simulink model "sampleModel197"  (R2021b)
settings: Solver=VariableStepAuto  StartTime=0.0  StopTime=10.0  RelTol=1e-3
undefined symbols (not defined in the file or in its folder): Newton, Raphson
libraries: simulink x2, slpidlib x1
settings Model: Creator=user  LastModifiedBy=user

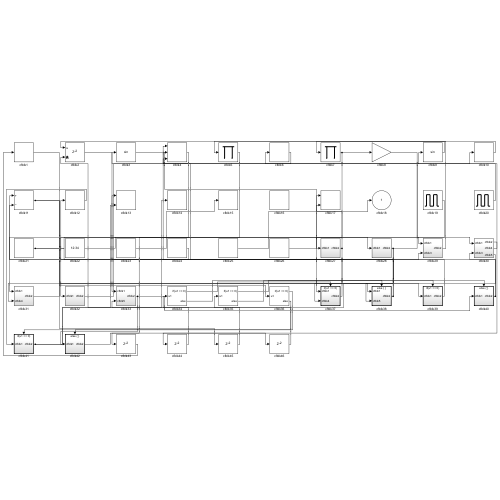
[thumbnail: Simulink's stored preview of the top-level diagram]
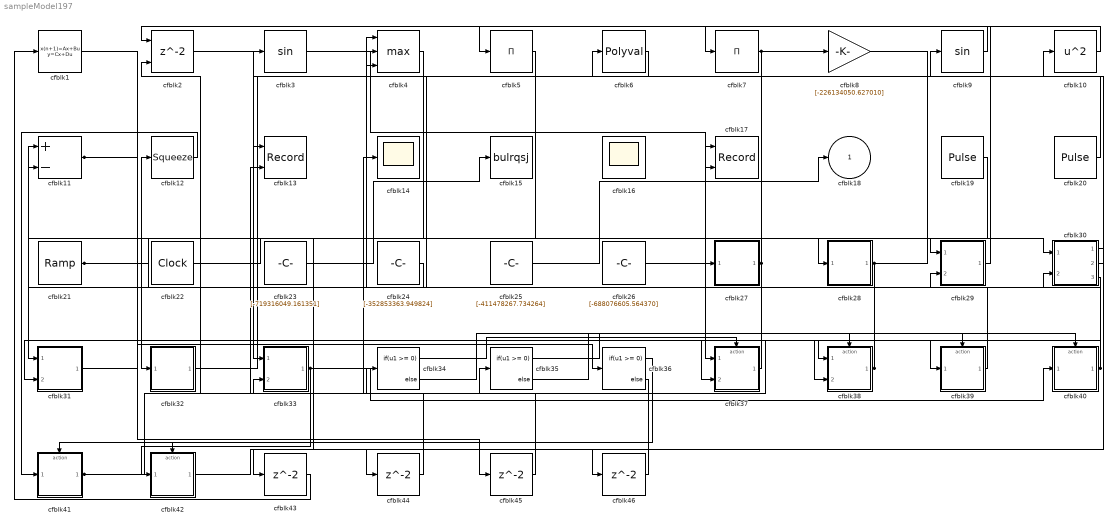
== system sampleModel197 ==
  cfblk1 : DiscreteStateSpace
  cfblk10 : Math  Operator=square  SaturateOnIntegerOverflow=on
  cfblk11 : Sum  Inputs=+-
  cfblk12 : Squeeze
  cfblk13 : Record  FileSettingsInternal="{\"entries\":[{\"content\":{\"excelSettings\":{\"content\":{},\"type\":\"Streamout.ExcelSettings\"}},\"type\":\"Streamout.FileSettingStorage\",\"uuid\":\"0279d5a8-bec8-47d0-96a9-0591946e5d00\"}],\"packageUris\":[\"http://schema.mathworks.com/mf0/streamout_blocks/R2020a\"],\"version\":\"1.0\"}"  Layout=[1 1]  SignalsInternal="{\"entries\":[{\"content\":{\"signals\":[{\"content\":{\"blockPath\":[\"sampleModel197/cfblk13\"],\"channel\":[],\"dimensions\":[1],\"domain\":\"sampleModel197/cfblk13\",\"lineColor\":\"#a2142f\",\"plots\":[1],\"port\":1,\"sid\":[\"\"],\"signalID\":7568,\"signalName\":\"cfblk40\"},\"type\":\"RecordBlkView.Signal\",\"uuid\":\"e7f566aa-51c7-4da6-b2fc-9a33eccfc797\"},{\"content\":{\"blockPath\":[\"sampleModel197/cfblk13\"],\"channel\":[],\"dimensions\":[1],\"domain\":\"sampleModel197/cfblk13\",\"lineColor\":\"#139fff\",\"plots\":[1],\"port\":2,\"sid\":[\"\"],\"signalID\":7572,\"signalName\":\"cfblk41\"},\"type\":\"RecordBlkView.Signal\",\"uuid\":\"1b39f455-c7ec-4c6a-a985-f4122d27351c\"}]},\"type\":\"RecordBlkView.InputSignals\",\"uuid\":\"b38396f4-be78-40d0-b78e-78bdf6d546fb\"}],\"packageUris\":[\"http://schema.mathworks.com/mf0/streamout_blocks/R2020a\"],\"version\":\"1.0\"}"  VisualizationBindings="{\"xyplotplugin\":{\"info\":[{\"series\":[{\"bindingParametersList\":[{\"parameter\":\"X-Axis\",\"signalID\":7568,\"signalName\":\"cfblk40\"},{\"parameter\":\"Y-Axis\",\"signalID\":7572,\"signalName\":\"cfblk41\"}],\"seriesID\":61193}],\"subplotID\":1}]}}"  CompatibilityTag=XY
  cfblk14 : Scope
  cfblk15 : ToWorkspace  VariableName=bulrqsj  SaveFormat=Timeseries  SampleTime=-1
  cfblk16 : Scope
      settings: Floating=on
  cfblk17 : Record  FileSettingsInternal="{\"entries\":[{\"content\":{\"excelSettings\":{\"content\":{},\"type\":\"Streamout.ExcelSettings\"}},\"type\":\"Streamout.FileSettingStorage\",\"uuid\":\"e6ae8cde-df67-4d7c-a82d-89148d2c1f8a\"}],\"packageUris\":[\"http://schema.mathworks.com/mf0/streamout_blocks/R2020a\"],\"version\":\"1.0\"}"  Layout=[1 1]  SignalsInternal="{\"entries\":[{\"content\":{\"signals\":[{\"content\":{\"blockPath\":[\"sampleModel197/cfblk17\"],\"channel\":[],\"dimensions\":[1],\"domain\":\"sampleModel197/cfblk17\",\"lineColor\":\"#a2142f\",\"plots\":[1],\"port\":1,\"sid\":[\"\"],\"signalID\":7576,\"signalName\":\"cfblk27\"},\"type\":\"RecordBlkView.Signal\",\"uuid\":\"cf26e29d-c82c-4e0b-80be-766500b7eef1\"},{\"content\":{\"blockPath\":[\"sampleModel197/cfblk17\"],\"channel\":[],\"dimensions\":[1],\"domain\":\"sampleModel197/cfblk17\",\"lineColor\":\"#139fff\",\"plots\":[1],\"port\":2,\"sid\":[\"\"],\"signalID\":7580,\"signalName\":\"cfblk26\"},\"type\":\"RecordBlkView.Signal\",\"uuid\":\"675d0609-db64-4a86-b5a2-412efc60ee90\"}]},\"type\":\"RecordBlkView.InputSignals\",\"uuid\":\"0deeecff-eec2-4d60-b210-f9e7a71af17f\"}],\"packageUris\":[\"http://schema.mathworks.com/mf0/streamout_blocks/R2020a\"],\"version\":\"1.0\"}"  VisualizationBindings="{\"xyplotplugin\":{\"info\":[{\"series\":[{\"bindingParametersList\":[{\"parameter\":\"X-Axis\",\"signalID\":7576,\"signalName\":\"cfblk27\"},{\"parameter\":\"Y-Axis\",\"signalID\":7580,\"signalName\":\"cfblk26\"}],\"seriesID\":48152}],\"subplotID\":1}]}}"  CompatibilityTag=XY
  cfblk19 : DiscretePulseGenerator  PulseType=Time based  Amplitude=[213944158.153628]  Period=[64533026.569931]  PulseWidth=5  PhaseDelay=[3.000000]
  cfblk2 : Delay  ShowEnablePort=on  SampleTime=1
      settings: InputPortMap=u0,e6
  cfblk20 : DiscretePulseGenerator  PulseType=Time based  Amplitude=[999071178.653989]  Period=[57734423.716283]  PulseWidth=5  PhaseDelay=[7.000000]
  cfblk21 : simulink/Sources/Ramp  slope=[-9275.531510]  start=[11.118864]  InitialOutput=[640340.774818]
  cfblk22 : DigitalClock
  cfblk23 : Constant  Value=[-719316049.161351]  SampleTime=1
  cfblk24 : Constant  Value=[-352853363.949824]  SampleTime=1
  cfblk25 : Constant  Value=[-411478267.734264]  SampleTime=1
  cfblk26 : Constant  Value=[-688076605.564370]  SampleTime=1
  cfblk27 : Subsystem
  cfblk28 : Subsystem
  cfblk29 : Subsystem
  cfblk3 : Trigonometry
  cfblk30 : Subsystem
  cfblk31 : Subsystem
  cfblk32 : Subsystem
  cfblk33 : Subsystem
  cfblk34 : If  IfExpression=u1 >= 0  SampleTime=1
  cfblk35 : If  IfExpression=u1 >= 0  SampleTime=1
  cfblk36 : If  IfExpression=u1 >= 0  SampleTime=1
  cfblk37 : Subsystem  TreatAsAtomicUnit=on
  cfblk38 : Subsystem  TreatAsAtomicUnit=on
  cfblk39 : Subsystem  TreatAsAtomicUnit=on
  cfblk4 : MinMax  Function=max  Inputs=3
  cfblk40 : Subsystem  TreatAsAtomicUnit=on
  cfblk41 : Subsystem  TreatAsAtomicUnit=on
  cfblk42 : Subsystem  TreatAsAtomicUnit=on
  cfblk{43..46} (4 alike) : Delay  SampleTime=1
  cfblk5 : Product  Inputs=*
  cfblk6 : Polyval  Coefs=[ +2.081618890e-019, -1.441693666e-014, +4.719686976e-010, -8.536869453e-006, +1.621573104e-001, -8.087801117e+001 ]
  cfblk7 : Product  Inputs=*
  cfblk8 : Gain  Gain=[-226134050.627010]
  cfblk9 : Trigonometry
  cfblk18 : Outport
  wires:
  cfblk23/1 -> cfblk15/1
  cfblk3/1 -> cfblk37/1(cfblk1)
  cfblk28/1(cfblk2) -> cfblk35/1, cfblk10/1, cfblk38/2(cfblk5)
  cfblk24/1 -> cfblk11/1
  cfblk33/1(cfblk2) -> cfblk40/1(cfblk1), cfblk42/1(cfblk1)
  cfblk37/1(cfblk2) -> cfblk11/2
  cfblk32/1(cfblk2) -> cfblk9/1
  cfblk11/1 -> cfblk36/1, cfblk45/1
  cfblk25/1 -> cfblk18/1
  cfblk2/1 -> cfblk33/1(cfblk1)
  cfblk7/1 -> cfblk8/1, cfblk31/1(cfblk1)
  cfblk27/1(cfblk2) -> cfblk17/1, cfblk31/2(cfblk4)
  cfblk12/1 -> cfblk41/1(cfblk1)
  cfblk29/1(cfblk2) -> cfblk5/1
  cfblk26/1 -> cfblk17/2
  cfblk10/1 -> cfblk7/1
  cfblk20/1 -> cfblk3/1
  cfblk39/1(cfblk2) -> cfblk4/1
  cfblk9/1 -> cfblk2/1
  cfblk5/1 -> cfblk32/1(cfblk1)
  cfblk21/1 -> cfblk29/1(cfblk1), cfblk29/2(cfblk3)
  cfblk41/1(cfblk2) -> cfblk14/1, cfblk13/2
  cfblk22/1 -> cfblk28/1(cfblk1)
  cfblk40/1(cfblk2) -> cfblk13/1, cfblk30/2(cfblk3)
  cfblk8/1 -> cfblk30/1(cfblk1)
  cfblk19/1 -> cfblk27/1(cfblk1)
  cfblk6/1 -> cfblk4/2
  cfblk1/1 -> cfblk39/1(cfblk1)
  cfblk30/2(cfblk4) -> cfblk6/1
  cfblk31/1(cfblk2) -> cfblk38/1(cfblk1)
  cfblk30/3(cfblk5) -> cfblk37/2(cfblk4)
  cfblk38/1(cfblk2) -> cfblk12/1, cfblk4/3
  cfblk34/1 -> cfblk37/Action
  cfblk34/2 -> cfblk38/Action
  cfblk35/1 -> cfblk39/Action
  cfblk35/2 -> cfblk40/Action
  cfblk36/1 -> cfblk41/Action
  cfblk36/2 -> cfblk42/Action
  cfblk4/1 -> cfblk43/1
  cfblk43/1 -> cfblk1/1
  cfblk30/1(cfblk2) -> cfblk44/1
  cfblk44/1 -> cfblk2/2
  cfblk45/1 -> cfblk34/1
  cfblk42/1(cfblk2) -> cfblk46/1
  cfblk46/1 -> cfblk33/2(cfblk5)

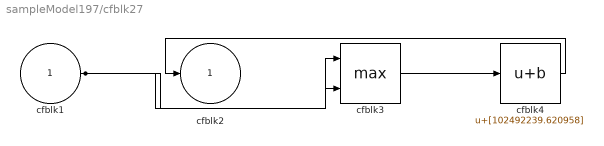
== system sampleModel197/cfblk27 ==
  cfblk1 : Inport
  cfblk3 : MinMax  Function=max  Inputs=2
  cfblk4 : Bias  Bias=[102492239.620958]
  cfblk2 : Outport
  wires:
  cfblk4/1 -> cfblk2/1
  cfblk3/1 -> cfblk4/1
  cfblk1/1 -> cfblk3/1, cfblk3/2

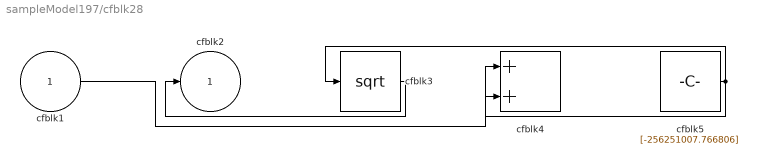
== system sampleModel197/cfblk28 ==
  cfblk1 : Inport
  cfblk3 : Sqrt  SaturateOnIntegerOverflow=on
  cfblk4 : Sum
  cfblk5 : Constant  Value=[-256251007.766806]  SampleTime=1
  cfblk2 : Outport
  wires:
  cfblk5/1 -> cfblk3/1, cfblk4/2
  cfblk3/1 -> cfblk2/1
  cfblk1/1 -> cfblk4/1

== system sampleModel197/cfblk29 ==
  cfblk1 : Inport
  cfblk3 : Inport  Port=2
  cfblk2 : Outport
  wires:
  cfblk1/1 -> cfblk2/1

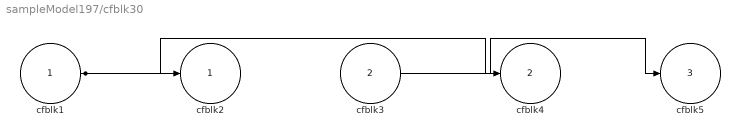
== system sampleModel197/cfblk30 ==
  cfblk1 : Inport
  cfblk3 : Inport  Port=2
  cfblk2 : Outport
  cfblk4 : Outport  Port=2
  cfblk5 : Outport  Port=3
  wires:
  cfblk3/1 -> cfblk5/1
  cfblk1/1 -> cfblk2/1, cfblk4/1

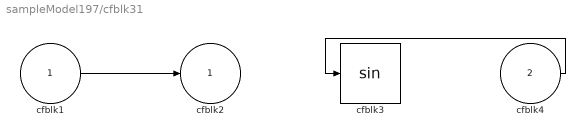
== system sampleModel197/cfblk31 ==
  cfblk1 : Inport
  cfblk4 : Inport  Port=2
  cfblk3 : Trigonometry
  cfblk2 : Outport
  wires:
  cfblk1/1 -> cfblk2/1
  cfblk4/1 -> cfblk3/1

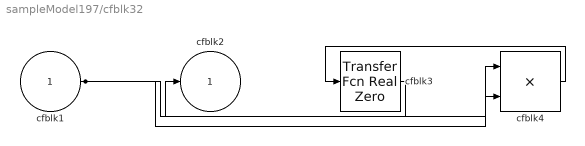
== system sampleModel197/cfblk32 ==
  cfblk1 : Inport
  cfblk3 : simulink/Discrete/Transfer Fcn Real Zero  ZeroZ=0.75  ICPrevInput=0.0  DoSatur=off
      settings: SourceProductBaseCode=SL
  cfblk4 : Product  Inputs=**
  cfblk2 : Outport
  wires:
  cfblk4/1 -> cfblk3/1
  cfblk3/1 -> cfblk2/1
  cfblk1/1 -> cfblk4/1, cfblk4/2

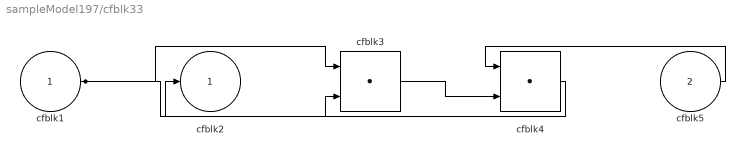
== system sampleModel197/cfblk33 ==
  cfblk1 : Inport
  cfblk5 : Inport  Port=2
  cfblk3 : DotProduct  InputSameDT=on  OutDataTypeStr=Inherit: Inherit via internal rule
  cfblk4 : DotProduct  InputSameDT=on  OutDataTypeStr=Inherit: Inherit via internal rule
  cfblk2 : Outport
  wires:
  cfblk5/1 -> cfblk4/1
  cfblk3/1 -> cfblk4/2
  cfblk4/1 -> cfblk2/1
  cfblk1/1 -> cfblk3/1, cfblk3/2

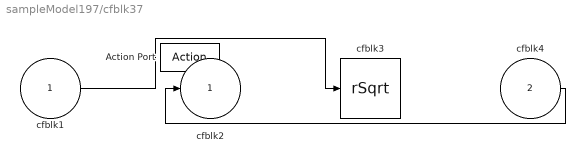
== system sampleModel197/cfblk37 ==
  cfblk1 : Inport
  cfblk4 : Inport  Port=2
  Action Port : ActionPort  ActionPortLabel=if(u1 >= 0)
  cfblk3 : Sqrt  Operator=rSqrt  AlgorithmType=Newton-Raphson  SaturateOnIntegerOverflow=on
  cfblk2 : Outport
  wires:
  cfblk4/1 -> cfblk2/1
  cfblk1/1 -> cfblk3/1

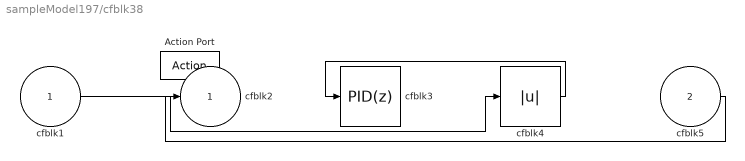
== system sampleModel197/cfblk38 ==
  cfblk1 : Inport
  cfblk5 : Inport  Port=2
  Action Port : ActionPort  ActionPortLabel=else
  cfblk3 : slpidlib/PID Controller  Controller=PID  Form=Parallel  TimeDomain=Discrete-time  UseExternalTs=off  SampleTime=-1  IntegratorMethod=Forward Euler  FilterMethod=Forward Euler  ControllerParametersSource=internal  P=1  I=1  D=0  UseFilter=on  N=100  TunerSelectOption=Transfer Function Based (PID Tuner App)  InitialConditionSource=internal  InitialConditionForIntegrator=0  InitialConditionForFilter=0  DifferentiatorICPrevScaledInput=0  ExternalReset=none  TrackingMode=off  Kt=1  LimitOutput=off  SatLimitsSource=internal  UpperSaturationLimit=inf  LowerSaturationLimit=-inf  LinearizeAsGain=off  AntiWindupMode=none  Kb=1  POutMin=[]  POutMax=[]  IOutMin=[]  IOutMax=[]  DOutMin=[]  DOutMax=[]  NOutMin=[]  NOutMax=[]  SumOutMin=[]  SumOutMax=[]  SaturationOutMin=[]  SaturationOutMax=[]  PParamMin=[]  PParamMax=[]  IParamMin=[]  IParamMax=[]  DParamMin=[]  DParamMax=[]  NParamMin=[]  NParamMax=[]  KbParamMin=[]  KbParamMax=[]  KtParamMin=[]  KtParamMax=[]  KbOutMin=[]  KbOutMax=[]  KtOutMin=[]  KtOutMax=[]  IntegratorOutMin=[]  IntegratorOutMax=[]  FilterOutMin=[]  FilterOutMax=[]  SumI1OutMin=[]  SumI1OutMax=[]  SumI2OutMin=[]  SumI2OutMax=[]  SumI3OutMin=[]  SumI3OutMax=[]  SumI4OutMin=[]  SumI4OutMax=[]  SumDOutMin=[]  SumDOutMax=[]  DifferentiatorOutMin=[]  DifferentiatorOutMax=[]  FilterDiffOutCoefMin=[]  FilterDiffOutCoefMax=[]  ReciprocalOutMin=[]  ReciprocalOutMax=[]  SumDenOutMin=[]  SumDenOutMax=[]  SumNumOutMin=[]  SumNumOutMax=[]  DivideOutMin=[]  DivideOutMax=[]  UdiffTsProdOutMin=[]  UdiffTsProdOutMax=[]  NTsProdOutMin=[]  NTsProdOutMax=[]  UintegralTsProdOutMin=[]  UintegralTsProdOutMax=[]  UngainTsProdOutMin=[]  UngainTsProdOutMax=[]  IntegratorContinuousStateAttributes=''  IntegratorStateMustResolveToSignalObject=off  IntegratorRTWStateStorageClass=Auto  FilterContinuousStateAttributes=''  FilterStateMustResolveToSignalObject=off  FilterRTWStateStorageClass=Auto  ParallelPVariant=InternalParameters  IdealPVariant=Disabled  IVariant=InternalParameters  DVariant=InternalParameters  IntegratorVariant=Discrete  SatVariant=Disabled  AWVariant=Passthrough  PCopyVariant=Disabled  TRVariant=Disabled  FdbkBlocksVariant=Forward  IdealPFdbkVariant=Disabled  SatFdbkVariant=Disabled  DerivativeFilterVariant=ForwardEulerFilter  NVariant=InternalParameters  NCopyVariant=Disabled  FilterICVariant=InternalICsFilter  IntegratorICVariant=InternalICs  ExternalResetVariant=Disabled  TRSumVariant=Passthrough  SumFdbkVariant=Disabled  SumVariant=Sum_PID  TsampFilterVariant=InternalTs  TsampNgainVariant=Passthrough  TsampIntegralVariant=Passthrough  ExternalSaturationOutDataTypeStr=Inherit: Same as second input
  cfblk4 : Abs
  cfblk2 : Outport
  wires:
  cfblk1/1 -> cfblk4/1
  cfblk5/1 -> cfblk2/1
  cfblk4/1 -> cfblk3/1

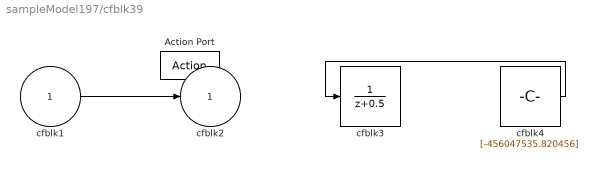
== system sampleModel197/cfblk39 ==
  cfblk1 : Inport
  Action Port : ActionPort  ActionPortLabel=if(u1 >= 0)
  cfblk3 : DiscreteTransferFcn
  cfblk4 : Constant  Value=[-456047535.820456]  SampleTime=1
  cfblk2 : Outport
  wires:
  cfblk1/1 -> cfblk2/1
  cfblk4/1 -> cfblk3/1

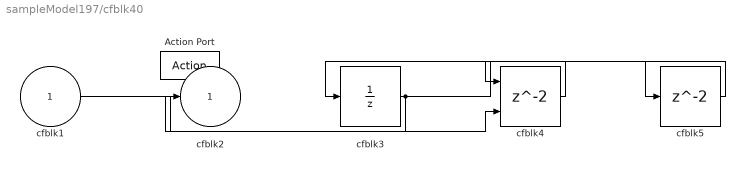
== system sampleModel197/cfblk40 ==
  cfblk1 : Inport
  Action Port : ActionPort  ActionPortLabel=else
  cfblk3 : UnitDelay  SampleTime=-1  HasFrameUpgradeWarning=on
  cfblk4 : Delay  ShowEnablePort=on
      settings: InputPortMap=u0,e6
  cfblk5 : Delay
  cfblk2 : Outport
  wires:
  cfblk3/1 -> cfblk2/1, cfblk5/1
  cfblk4/1 -> cfblk3/1
  cfblk1/1 -> cfblk4/2
  cfblk5/1 -> cfblk4/1

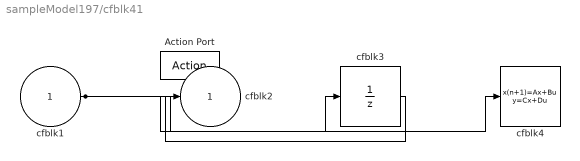
== system sampleModel197/cfblk41 ==
  cfblk1 : Inport
  Action Port : ActionPort  ActionPortLabel=if(u1 >= 0)
  cfblk3 : UnitDelay  SampleTime=-1  HasFrameUpgradeWarning=on
  cfblk4 : DiscreteStateSpace  SampleTime=-1
  cfblk2 : Outport
  wires:
  cfblk1/1 -> cfblk3/1, cfblk4/1
  cfblk3/1 -> cfblk2/1

== system sampleModel197/cfblk42 ==
  cfblk1 : Inport
  Action Port : ActionPort  ActionPortLabel=else
  cfblk3 : Delay  ShowEnablePort=on
      settings: InputPortMap=u0,e6
  cfblk2 : Outport
  wires:
  cfblk1/1 -> cfblk2/1, cfblk3/1, cfblk3/2
